simulink model "turbine"  (R2020b)
settings: Solver=VariableStepAuto  StartTime=0.0  StopTime=1  RelTol=1e-3
libraries: powerlib x1
settings Model: Creator=a6039  LastModifiedBy=axz5845

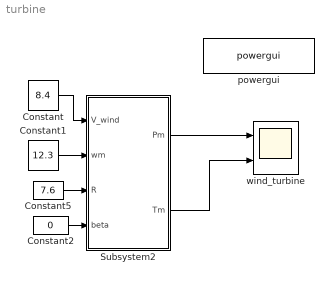
== system turbine ==
  Constant : Constant  Value=8.4
  Constant1 : Constant  Value=12.3
  Constant2 : Constant  Value=0
  Constant5 : Constant  Value=7.6
  Subsystem2 : Subsystem
  powergui : powerlib/powergui  Priority=1  SimulationMode=Discrete  SampleTime=5e-6  frequency=60  Iterations=50  frequencyindice=0  Pbase=100e6  ErrMax=1e-4  UnitsV=kV  UnitsW=MW  buscounter=0  FunctionMessages=off  echomessages=off  EnableUseOfTLC=off  CurrentSourceSwitches=off  DisableSnubberDevices=off  DisableRonSwitches=off  DisableVfSwitches=off  DisplayEquations=off  AutomaticDiscreteSolvers=off  SolverType=Tustin  Interpol=off  ExternalGateDelay=off  methode=off  Ts=0  x0status=blocks  SPID=off  SwTol=0  HookPort=off  NonlinearTolerance=1e-4  nMaxIteration=100  ContinueOnMaxIteration=off  RestoreLinks=warning  ResistiveCurrentMeasurement=off  Frange=[0:2:500]  Ylog=off  Xlog=on  ShowGrid=off  save=off  variable=ZData  structure=voltage_and_current  ZoomFFT=off  StartTime=1.5  cycles=3  DisplayStyle=3  fundamental=50  FreqAxis=on  MaxFrequency=2000  frequencyindicesteady=1  RmsSteady=1  display=off
  wind_turbine : Scope  NumInputPorts=2
  wires:
  Constant/1 -> Subsystem2/1(V_wind)
  Constant5/1 -> Subsystem2/3(R)
  Subsystem2/2(Tm) -> wind_turbine/2
  Subsystem2/1(Pm) -> wind_turbine/1
  Constant2/1 -> Subsystem2/4(beta)
  Constant1/1 -> Subsystem2/2(wm)

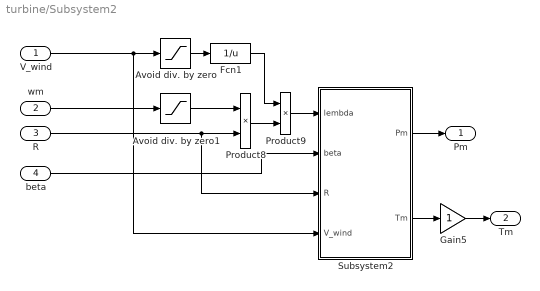
== system turbine/Subsystem2 ==
  V_wind : Inport
  wm : Inport  Port=2
  R : Inport  Port=3
  beta : Inport  Port=4
  Avoid div. by zero : Saturate  UpperLimit=inf  LowerLimit=eps
  Avoid div. by zero1 : Saturate  UpperLimit=inf  LowerLimit=eps
  Fcn1 : Fcn  Expr=1/u
  Gain5 : Gain
  Product8 : Product  RndMeth=Zero
  Product9 : Product  RndMeth=Zero
  Subsystem2 : Subsystem
  Pm : Outport  VectorParamsAs1DForOutWhenUnconnected=off
  Tm : Outport  Port=2  VectorParamsAs1DForOutWhenUnconnected=off
  wires:
  Product9/1 -> Subsystem2/1(lembda)
  V_wind/1 -> Subsystem2/4(V_wind), Avoid div. by zero/1
  Avoid div. by zero/1 -> Fcn1/1
  Product8/1 -> Product9/2
  Fcn1/1 -> Product9/1
  R/1 -> Product8/2, Subsystem2/3(R)
  wm/1 -> Avoid div. by zero1/1
  Subsystem2/2(Tm) -> Gain5/1
  beta/1 -> Subsystem2/2(beta)
  Gain5/1 -> Tm/1
  Subsystem2/1(Pm) -> Pm/1
  Avoid div. by zero1/1 -> Product8/1

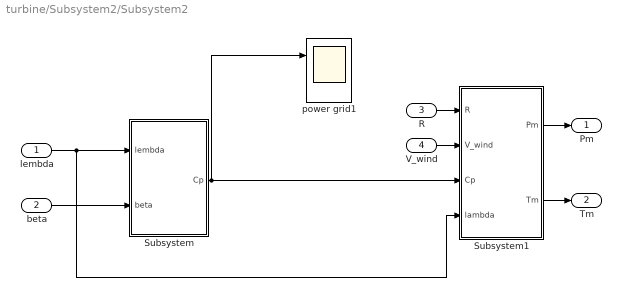
== system turbine/Subsystem2/Subsystem2 ==
  lembda : Inport
  beta : Inport  Port=2
  R : Inport  Port=3
  V_wind : Inport  Port=4
  Subsystem : Subsystem  mask{c1=0.5176, c2=116, c3=0.4, c4=5, c5=21, c6=0.0068}
  Subsystem1 : Subsystem
  power grid1 : Scope  NumInputPorts=2
  Pm : Outport  VectorParamsAs1DForOutWhenUnconnected=off
  Tm : Outport  Port=2  VectorParamsAs1DForOutWhenUnconnected=off
  wires:
  lembda/1 -> Subsystem1/4(lambda), Subsystem/1(lembda)
  beta/1 -> Subsystem/2(beta)
  R/1 -> Subsystem1/1(R)
  Subsystem1/1(Pm) -> Pm/1
  Subsystem1/2(Tm) -> Tm/1
  V_wind/1 -> Subsystem1/2(V_wind)
  Subsystem/1(Cp) -> power grid1/1, Subsystem1/3(Cp)

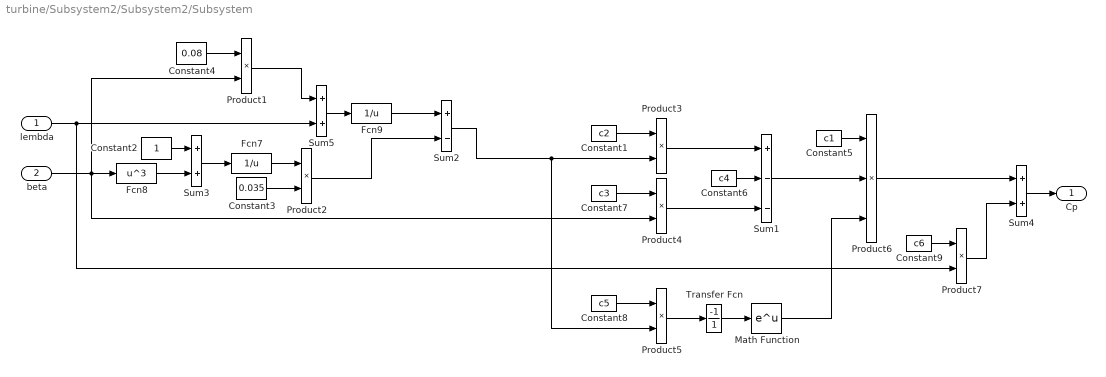
== system turbine/Subsystem2/Subsystem2/Subsystem ==
  lembda : Inport
  beta : Inport  Port=2
  Constant1 : Constant  Value=c2
  Constant2 : Constant
  Constant3 : Constant  Value=0.035
  Constant4 : Constant  Value=0.08
  Constant5 : Constant  Value=c1
  Constant6 : Constant  Value=c4
  Constant7 : Constant  Value=c3
  Constant8 : Constant  Value=c5
  Constant9 : Constant  Value=c6
  Fcn7 : Fcn  Expr=1/u
  Fcn8 : Fcn  Expr=u^3
  Fcn9 : Fcn  Expr=1/u
  Math Function : Math  SignedPower=on  SaturateOnIntegerOverflow=on
  Product{1..5,7} (6 alike) : Product  RndMeth=Zero
  Product6 : Product  Inputs=3  RndMeth=Zero
  Sum1 : Sum  Inputs=+--
  Sum2 : Sum  Inputs=+-
  Sum3 : Sum
  Sum4 : Sum
  Sum5 : Sum
  Transfer Fcn : TransferFcn  Numerator=[-1]  Denominator=[1]
  Cp : Outport  VectorParamsAs1DForOutWhenUnconnected=off
  wires:
  Product6/1 -> Sum4/1
  Product7/1 -> Sum4/2
  Constant9/1 -> Product7/1
  Math Function/1 -> Product6/3
  Constant5/1 -> Product6/1
  Sum1/1 -> Product6/2
  Transfer Fcn/1 -> Math Function/1
  Product5/1 -> Transfer Fcn/1
  Constant8/1 -> Product5/1
  Product4/1 -> Sum1/3
  Constant6/1 -> Sum1/2
  Constant7/1 -> Product4/1
  Product3/1 -> Sum1/1
  Constant1/1 -> Product3/1
  Sum2/1 -> Product3/2, Product5/2
  Sum5/1 -> Fcn9/1
  lembda/1 -> Product7/2, Sum5/2
  Product1/1 -> Sum5/1
  Constant4/1 -> Product1/1
  Product2/1 -> Sum2/2
  Constant3/1 -> Product2/2
  Fcn7/1 -> Product2/1
  Fcn8/1 -> Sum3/2
  Sum3/1 -> Fcn7/1
  beta/1 -> Product1/2, Fcn8/1, Product4/2
  Constant2/1 -> Sum3/1
  Fcn9/1 -> Sum2/1
  Sum4/1 -> Cp/1

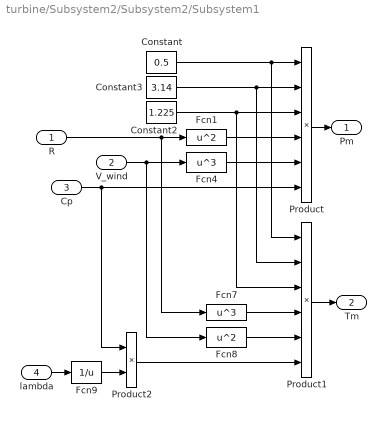
== system turbine/Subsystem2/Subsystem2/Subsystem1 ==
  R : Inport
  V_wind : Inport  Port=2
  Cp : Inport  Port=3
  lambda : Inport  Port=4
  Constant : Constant  Value=0.5
  Constant2 : Constant  Value=1.225
  Constant3 : Constant  Value=3.14
  Fcn1 : Fcn  Expr=u^2
  Fcn4 : Fcn  Expr=u^3
  Fcn7 : Fcn  Expr=u^3
  Fcn8 : Fcn  Expr=u^2
  Fcn9 : Fcn  Expr=1/u
  Product : Product  Inputs=6  RndMeth=Zero
  Product1 : Product  Inputs=6  RndMeth=Zero
  Product2 : Product  RndMeth=Zero
  Pm : Outport  VectorParamsAs1DForOutWhenUnconnected=off
  Tm : Outport  Port=2  VectorParamsAs1DForOutWhenUnconnected=off
  wires:
  R/1 -> Fcn7/1, Fcn1/1
  V_wind/1 -> Fcn8/1, Fcn4/1
  Constant/1 -> Product/1, Product1/1
  Constant3/1 -> Product/2, Product1/2
  Constant2/1 -> Product/3, Product1/3
  Fcn1/1 -> Product/4
  Fcn4/1 -> Product/5
  Cp/1 -> Product2/1, Product/6
  Fcn7/1 -> Product1/4
  Fcn8/1 -> Product1/5
  Fcn9/1 -> Product2/2
  Product2/1 -> Product1/6
  Product/1 -> Pm/1
  Product1/1 -> Tm/1
  lambda/1 -> Fcn9/1
